simulink model "kongzhi"  (R2023a)
settings: Solver=ode23tb  StartTime=0.0  StopTime=0.5  RelTol=1e-3
libraries: spsAsynchronousMachineSIUnitsLib x1, spsDCVoltageSourceLib x1, spsGroundLib x1, spsThreePhaseVIMeasurementLib x1, spsUniversalBridgeLib x1, sps_lib x1
settings Model: Creator=ASUS  LastModifiedBy=ASUS

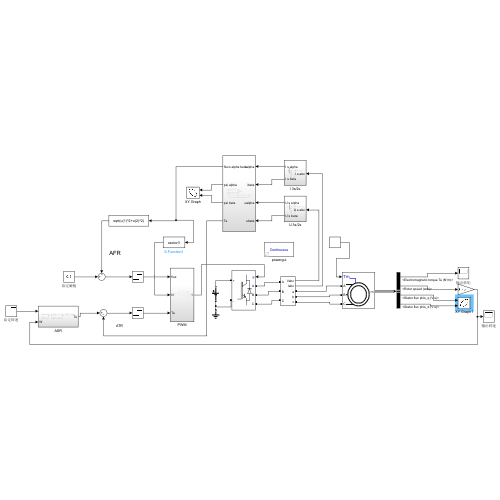
[thumbnail: Simulink's stored preview of the top-level diagram]
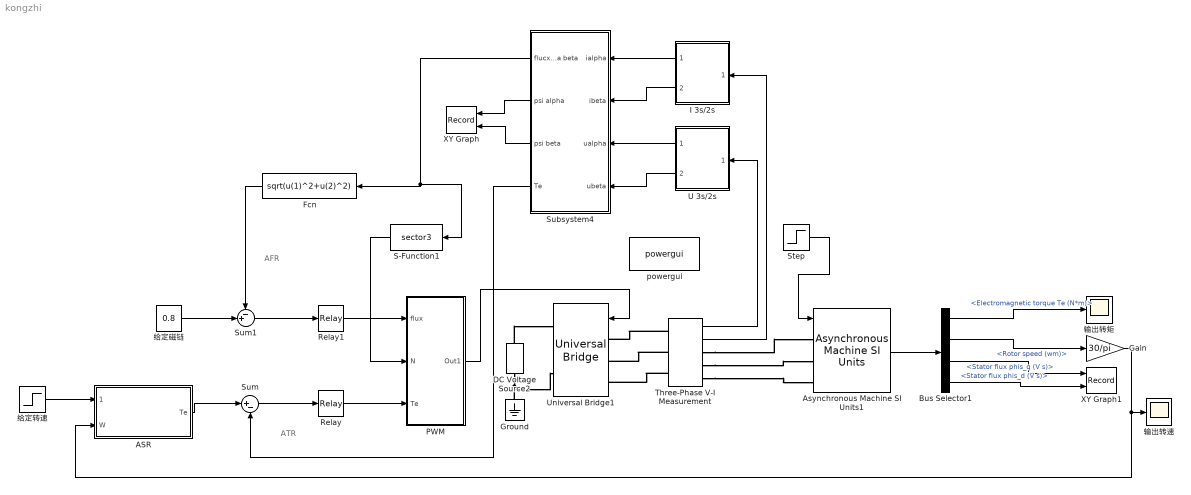
== system kongzhi ==
  note: ATR
  note: AFR
  ASR : Subsystem
  Asynchronous Machine SI Units1 : spsAsynchronousMachineSIUnitsLib/Asynchronous Machine SI Units  RotorType=Squirrel-cage  PresetModel="17:  20 HP (15KW)   400 V 50Hz 1460 RPM"  MechanicalLoad=Torque Tm  ShowDetailedParameters=on  ReferenceFrame=Stationary  Units=SI  MeasurementBus=off  NominalParameters=[1.5e+04 400 50]  VoltageRatio=1  Stator=[0.2147 0.000991]  Rotor=[0.2205 0.000991]  Cage1=[ 0.022 0.226/377]  Cage2=[ 0.022 0.226/377]  Lm=0.06419  Mechanical=[0.102 0.009541 2]  PolePairs=2  InitialConditions="[ 1,0   0,0,0   0,0,0 ]"  SimulateSaturation=off  Saturation=[9.9249,19.6672,38.0377,51.3988,69.2824,105.1337,152.5532,214.2421,303.1917;230, 322, 414, 460, 506, 552, 598, 644, 690]  LoadFlowParameters=0  TsPowergui=0  TsBlock=-1  IterativeModel=Forward Euler  IterativeDiscreteModel=Trapezoidal non iterative  Pmec=0
  Bus Selector1 : BusSelector  OutputSignals=Mechanical.Electromagnetic torque Te (N*m),Mechanical.Rotor speed (wm),Stator measurements.Stator flux phis_q (V s),Stator measurements.Stator flux phis_d (V s)
  DC Voltage Source2 : spsDCVoltageSourceLib/DC Voltage Source  Amplitude=400  Measurements=None
  Fcn : Fcn  Expr=sqrt(u(1)^2+u(2)^2)
  Gain : Gain  Gain=30/pi
  Ground : spsGroundLib/Ground  LConnTagsString=a
  I 3s/2s : Subsystem
  PWM : Subsystem
  Relay : Relay  OnSwitchValue=0.5  OffSwitchValue=-0.5
  Relay1 : Relay  OnSwitchValue=0.001  OffSwitchValue=-0.001
  S-Function1 : S-Function  FunctionName=sector3  SFunctionDeploymentMode=off  EnableBusSupport=off
  Step : Step  Time=0  Before=50  After=50  SampleTime=0
  Subsystem4 : Subsystem
  Sum : Sum  Inputs=|+-
  Sum1 : Sum  Inputs=-+|
  Three-Phase V-I Measurement : spsThreePhaseVIMeasurementLib/Three-Phase V-I Measurement  VoltageMeasurement=phase-to-ground  SetLabelV=off  LabelV=Vabc  Vpu=off  VpuLL=off  CurrentMeasurement=yes  SetLabelI=off  LabelI=Iabc  Ipu=off  Pbase=100e6  Vbase=500e3  OutputType=Complex  PhasorSimulation=off  PSBequivalent=0
  U 3s/2s : Subsystem
  Universal Bridge1 : spsUniversalBridgeLib/Universal Bridge  Arms=3  SnubberResistance=1e5  SnubberCapacitance=inf  Device=IGBT / Diodes  Ron=1e-3  Lon=0  ForwardVoltages="[  0  0  ]"  ForwardVoltage=0  GTOparameters=[ 10e-6 , 20e-6 ]  IGBTparameters=[ 1e-6 , 2e-6 ]  Measurements=None  Measurements_2=None  converterType=Rectifier
  XY Graph : Record  FileSettingsInternal="{\"entries\":[{\"content\":{\"excelSettings\":{\"content\":{},\"type\":\"Streamout.ExcelSettings\"}},\"type\":\"Streamout.FileSettingStorage\",\"uuid\":\"d99a5585-4551-4ee5-a23c-574eb21537c6\"}],\"packageUris\":[\"http://schema.mathworks.com/mf0/streamout_blocks/R2020a\"],\"version\":\"1.0\"}"  Layout=[1 1]  SignalsInternal="{\"entries\":[{\"content\":{\"signals\":[{\"content\":{\"blockPath\":[\"kongzhi/XY Graph\"],\"dimensions\":[1],\"domain\":\"kongzhi/XY Graph\",\"lineColor\":\"#a2142f\",\"plots\":[1],\"port\":1,\"sid\":[\"\"],\"signalID\":22656,\"signalName\":\"Subsystem4:2\"},\"type\":\"RecordBlkView.Signal\",\"uuid\":\"df6e7023-f9b9-436d-a626-336ee013b6ea\"},{\"content\":{\"blockPath\":[\"kongzhi/XY Graph\"],\"dimensions\":[1],\"domain\":\"kongzhi/XY Graph\",\"lineColor\":\"#139fff\",\"plots\":[1],\"port\":2,\"sid\":[\"\"],\"signalID\":22660,\"signalName\":\"Subsystem4:3\"},\"type\":\"RecordBlkView.Signal\",\"uuid\":\"d19e1cbc-f2ff-4bfc-97e4-62be1705afae\"}]},\"type\":\"RecordBlkView.InputSignals\",\"uuid\":\"3aea963f-f125-4d09-981d-9f07b36c2ba5\"}],\"packageUris\":[\"http://schema.mathworks.com/mf0/streamout_blocks/R2020a\"],\"version\":\"1.0\"}"  VisualizationBindings="{\"xyplotplugin\":{\"info\":[{\"series\":[{\"bindingParametersList\":[{\"parameter\":\"X-Axis\",\"signalID\":22656,\"signalName\":\"Subsystem4:2\"},{\"parameter\":\"Y-Axis\",\"signalID\":22660,\"signalName\":\"Subsystem4:3\"}],\"seriesID\":30182}],\"subplotID\":1}]}}"  CompatibilityTag=XY
  XY Graph1 : Record  FileSettingsInternal="{\"entries\":[{\"content\":{\"excelSettings\":{\"content\":{},\"type\":\"Streamout.ExcelSettings\"}},\"type\":\"Streamout.FileSettingStorage\",\"uuid\":\"2f48a670-b858-471d-9210-6afec38b2273\"}],\"packageUris\":[\"http://schema.mathworks.com/mf0/streamout_blocks/R2020a\"],\"version\":\"1.0\"}"  Layout=[1 1]  SignalsInternal="{\"entries\":[{\"content\":{\"signals\":[{\"content\":{\"blockPath\":[\"kongzhi/XY Graph1\"],\"dimensions\":[1],\"domain\":\"kongzhi/XY Graph1\",\"lineColor\":\"#a2142f\",\"plots\":[1],\"port\":1,\"sid\":[\"\"],\"signalID\":22664,\"signalName\":\"<Stator flux phis_q (V s)>\"},\"type\":\"RecordBlkView.Signal\",\"uuid\":\"a525e989-c708-4338-98a2-6f3b374b03e2\"},{\"content\":{\"blockPath\":[\"kongzhi/XY Graph1\"],\"dimensions\":[1],\"domain\":\"kongzhi/XY Graph1\",\"lineColor\":\"#139fff\",\"plots\":[1],\"port\":2,\"sid\":[\"\"],\"signalID\":22668,\"signalName\":\"<Stator flux phis_d (V s)>\"},\"type\":\"RecordBlkView.Signal\",\"uuid\":\"1f8a1f75-314e-4074-bfd5-83f112e8ba22\"}]},\"type\":\"RecordBlkView.InputSignals\",\"uuid\":\"839f365b-2055-442e-9575-d9756f1278d4\"}],\"packageUris\":[\"http://schema.mathworks.com/mf0/streamout_blocks/R2020a\"],\"version\":\"1.0\"}"  VisualizationBindings="{\"xyplotplugin\":{\"info\":[{\"series\":[{\"bindingParametersList\":[{\"parameter\":\"X-Axis\",\"signalID\":22664,\"signalName\":\"<Stator flux phis_q (V s)>\"},{\"parameter\":\"Y-Axis\",\"signalID\":22668,\"signalName\":\"<Stator flux phis_d (V s)>\"}],\"seriesID\":31724}],\"subplotID\":1}]}}"  CompatibilityTag=XY
  powergui : sps_lib/powergui  Priority=1  SimulationMode=Continuous  SampleTime=50e-6  frequency=60  Iterations=50  frequencyindice=50  Pbase=100e6  ErrMax=1e-4  UnitsV=kV  UnitsW=MW  buscounter=0  FunctionMessages=off  echomessages=off  EnableUseOfTLC=off  CurrentSourceSwitches=off  DisableSnubberDevices=off  DisableRonSwitches=off  DisableVfSwitches=off  DisplayEquations=off  AutomaticDiscreteSolvers=off  SolverType=Tustin/Backward Euler (TBE)  Interpol=off  ExternalGateDelay=off  methode=off  Ts=100  x0status=blocks  SPID=on  SwTol=0  HookPort=off  NonlinearTolerance=1e-4  nMaxIteration=100  ContinueOnMaxIteration=off  RestoreLinks=warning  ResistiveCurrentMeasurement=off  Frange=[0:2:500]  Ylog=off  Xlog=on  ShowGrid=off  save=off  variable=ZData  structure=0  ZoomFFT=off  StartTime=0.0  cycles=1  DisplayStyle=1  fundamental=60  FreqAxis=off  MaxFrequency=1000  frequencyindicesteady=1  RmsSteady=1  display=off
  给定磁链 : Constant  Value=0.8
  给定转速 : Step  Time=0  Before=1000  After=1000  SampleTime=0  VectorParams1D=off
  输出转矩 : Scope
  输出转速 : Scope
  wires:
  Asynchronous Machine SI Units1/1 -> Bus Selector1/1
  给定转速/1 -> ASR/1(" ")
  Bus Selector1/2 -> Gain/1  "<Rotor speed (wm)>"
  Gain/1 -> ASR/2(W), 输出转速/1
  ASR/1(Te) -> Sum/1
  Sum/1 -> Relay/1
  Sum1/1 -> Relay1/1
  Relay1/1 -> PWM/1(flux)
  Relay/1 -> PWM/3(Te)
  S-Function1/1 -> PWM/2(N)
  PWM/1(Out1) -> Universal Bridge1/1
  Three-Phase V-I Measurement/2 -> I 3s/2s/1(I s abc)
  Three-Phase V-I Measurement/1 -> U 3s/2s/1(U s abc)
  I 3s/2s/1(I s alpha) -> Subsystem4/1(ialpha)
  I 3s/2s/2(I s beta) -> Subsystem4/2(ibeta)
  U 3s/2s/1(U s alpha) -> Subsystem4/3(ualpha)
  U 3s/2s/2(U s beta) -> Subsystem4/4(ubeta)
  Subsystem4/2(psi alpha) -> XY Graph/1
  Subsystem4/3(psi beta) -> XY Graph/2
  Subsystem4/1(flucx alpha beta) -> S-Function1/1, Fcn/1
  给定磁链/1 -> Sum1/2
  Fcn/1 -> Sum1/1
  Subsystem4/4(Te) -> Sum/2
  Bus Selector1/1 -> 输出转矩/1  "<Electromagnetic torque Te (N*m)>"
  Step/1 -> Asynchronous Machine SI Units1/1
  Bus Selector1/3 -> XY Graph1/1  "<Stator flux phis_q (V s)>"
  Bus Selector1/4 -> XY Graph1/2  "<Stator flux phis_d (V s)>"
  connections:
  DC Voltage Source2/LConn1 -- Universal Bridge1/RConn2 -- Ground/LConn1
  DC Voltage Source2/RConn1 -- Universal Bridge1/RConn1
  Three-Phase V-I Measurement/LConn1 -- Universal Bridge1/LConn1
  Three-Phase V-I Measurement/LConn2 -- Universal Bridge1/LConn2
  Three-Phase V-I Measurement/LConn3 -- Universal Bridge1/LConn3
  Three-Phase V-I Measurement/RConn2 -- Asynchronous Machine SI Units1/LConn2
  Three-Phase V-I Measurement/RConn3 -- Asynchronous Machine SI Units1/LConn3
  Three-Phase V-I Measurement/RConn1 -- Asynchronous Machine SI Units1/LConn1

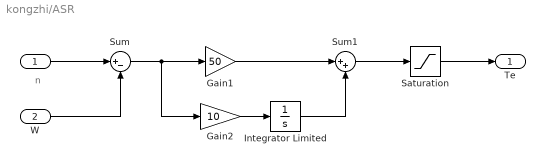
== system kongzhi/ASR ==
  note: n
  " " : Inport
  W : Inport  Port=2
  Gain1 : Gain  Gain=50
  Gain2 : Gain  Gain=10  OutMin=[-200]  OutMax=[200]
  Integrator Limited : Integrator  LimitOutput=on  UpperSaturationLimit=120  LowerSaturationLimit=-120
  Saturation : Saturate  UpperLimit=120  LowerLimit=-120
  Sum : Sum  Inputs=|+-
  Sum1 : Sum  Inputs=|++
  Te : Outport  VectorParamsAs1DForOutWhenUnconnected=off
  wires:
  Integrator Limited/1 -> Sum1/2
  " "/1 -> Sum/1
  Gain1/1 -> Sum1/1
  Sum/1 -> Gain2/1, Gain1/1
  Gain2/1 -> Integrator Limited/1
  Sum1/1 -> Saturation/1
  W/1 -> Sum/2
  Saturation/1 -> Te/1

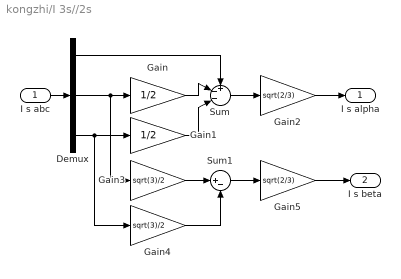
== system kongzhi/I 3s//2s ==
  I s abc : Inport
  Demux : Demux  Outputs=3
  Gain : Gain  Gain=1/2
  Gain1 : Gain  Gain=1/2
  Gain2 : Gain  Gain=sqrt(2/3)
  Gain3 : Gain  Gain=sqrt(3)/2
  Gain4 : Gain  Gain=sqrt(3)/2
  Gain5 : Gain  Gain=sqrt(2/3)
  Sum : Sum  Inputs=+--|
  Sum1 : Sum  Inputs=|+-
  I s alpha : Outport  VectorParamsAs1DForOutWhenUnconnected=off
  I s beta : Outport  Port=2  VectorParamsAs1DForOutWhenUnconnected=off
  wires:
  I s abc/1 -> Demux/1
  Demux/1 -> Sum/1
  Demux/3 -> Gain4/1, Gain1/1
  Demux/2 -> Gain3/1, Gain/1
  Sum/1 -> Gain2/1
  Gain2/1 -> I s alpha/1
  Gain3/1 -> Sum1/1
  Gain4/1 -> Sum1/2
  Sum1/1 -> Gain5/1
  Gain/1 -> Sum/2
  Gain1/1 -> Sum/3
  Gain5/1 -> I s beta/1

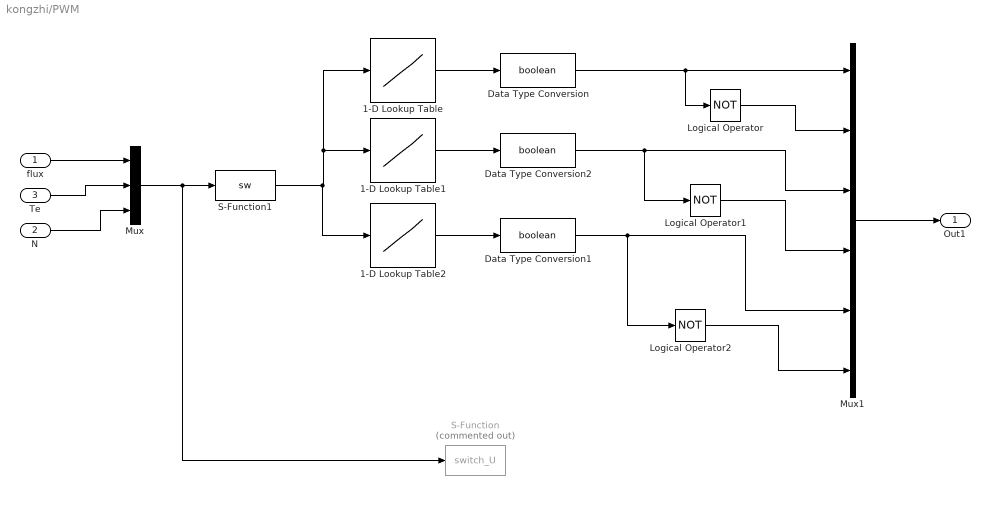
== system kongzhi/PWM ==
  flux : Inport
  N : Inport  Port=2
  Te : Inport  Port=3
  1-D Lookup Table : Lookup_n-D  NumberOfTableDimensions=1  BreakpointsForDimension1=[1 2 3 4 5 6]  Table=[1 1 1 0 0 0]  InternalRulePriority=Speed  RndMeth=Simplest
  1-D Lookup Table1 : Lookup_n-D  NumberOfTableDimensions=1  BreakpointsForDimension1=[1 2 3 4 5 6]  Table=[1 0 0 1 1 0]  InternalRulePriority=Speed  RndMeth=Simplest
  1-D Lookup Table2 : Lookup_n-D  NumberOfTableDimensions=1  BreakpointsForDimension1=[1 2 3 4 5 6]  Table=[0 1 0 1 0 1]  InternalRulePriority=Speed  RndMeth=Simplest
  Data Type Conversion : DataTypeConversion  OutDataTypeStr=boolean  SaturateOnIntegerOverflow=off  RndMeth=Floor
  Data Type Conversion1 : DataTypeConversion  OutDataTypeStr=boolean  SaturateOnIntegerOverflow=off  RndMeth=Floor
  Data Type Conversion2 : DataTypeConversion  OutDataTypeStr=boolean  SaturateOnIntegerOverflow=off  RndMeth=Floor
  Logical Operator : Logic  Operator=NOT  AllPortsSameDT=off  OutDataTypeStr=boolean
  Logical Operator1 : Logic  Operator=NOT  AllPortsSameDT=off  OutDataTypeStr=boolean
  Logical Operator2 : Logic  Operator=NOT  AllPortsSameDT=off  OutDataTypeStr=boolean
  Mux : Mux  Inputs=3
  Mux1 : Mux  Inputs=6
  S-Function : S-Function  Commented=on  FunctionName=switch_U  SFunctionDeploymentMode=off  EnableBusSupport=off
  S-Function1 : S-Function  FunctionName=sw  SFunctionDeploymentMode=off  EnableBusSupport=off
  Out1 : Outport
  wires:
  flux/1 -> Mux/1
  Te/1 -> Mux/2
  N/1 -> Mux/3
  S-Function1/1 -> 1-D Lookup Table2/1, 1-D Lookup Table1/1, 1-D Lookup Table/1
  1-D Lookup Table/1 -> Data Type Conversion/1
  1-D Lookup Table1/1 -> Data Type Conversion2/1
  1-D Lookup Table2/1 -> Data Type Conversion1/1
  Data Type Conversion/1 -> Logical Operator/1, Mux1/1
  Logical Operator/1 -> Mux1/2
  Data Type Conversion2/1 -> Logical Operator1/1, Mux1/3
  Logical Operator1/1 -> Mux1/4
  Data Type Conversion1/1 -> Logical Operator2/1, Mux1/5
  Logical Operator2/1 -> Mux1/6
  Mux/1 -> S-Function/1, S-Function1/1
  Mux1/1 -> Out1/1

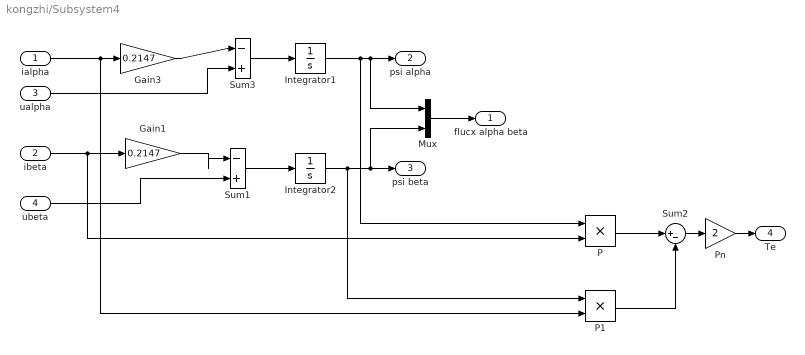
== system kongzhi/Subsystem4 ==
  ialpha : Inport
  ibeta : Inport  Port=2
  ualpha : Inport  Port=3
  ubeta : Inport  Port=4
  Gain1 : Gain  Gain=0.2147
  Gain3 : Gain  Gain=0.2147
  Integrator1 : Integrator
  Integrator2 : Integrator
  Mux : Mux  Inputs=2
  P : Product  Inputs=**
  P1 : Product  Inputs=**
  Pn : Gain  Gain=2
  Sum1 : Sum  Inputs=|-+
  Sum2 : Sum  Inputs=|+-
  Sum3 : Sum  Inputs=|-+
  flucx alpha beta : Outport
  psi alpha : Outport  Port=2
  psi beta : Outport  Port=3
  Te : Outport  Port=4  VectorParamsAs1DForOutWhenUnconnected=off
  wires:
  ialpha/1 -> P1/2, Gain3/1
  Gain3/1 -> Sum3/1
  ualpha/1 -> Sum3/2
  ubeta/1 -> Sum1/2
  ibeta/1 -> P/2, Gain1/1
  Gain1/1 -> Sum1/1
  Sum3/1 -> Integrator1/1
  Sum1/1 -> Integrator2/1
  Integrator1/1 -> P/1, Mux/1, psi alpha/1
  Mux/1 -> flucx alpha beta/1
  P/1 -> Sum2/1
  P1/1 -> Sum2/2
  Sum2/1 -> Pn/1
  Pn/1 -> Te/1
  Integrator2/1 -> P1/1, psi beta/1, Mux/2

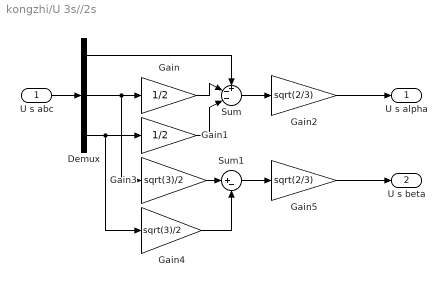
== system kongzhi/U 3s//2s ==
  U s abc : Inport
  Demux : Demux  Outputs=3
  Gain : Gain  Gain=1/2
  Gain1 : Gain  Gain=1/2
  Gain2 : Gain  Gain=sqrt(2/3)
  Gain3 : Gain  Gain=sqrt(3)/2
  Gain4 : Gain  Gain=sqrt(3)/2
  Gain5 : Gain  Gain=sqrt(2/3)
  Sum : Sum  Inputs=+--|
  Sum1 : Sum  Inputs=|+-
  U s alpha : Outport  VectorParamsAs1DForOutWhenUnconnected=off
  U s beta : Outport  Port=2  VectorParamsAs1DForOutWhenUnconnected=off
  wires:
  Demux/3 -> Gain4/1, Gain1/1
  U s abc/1 -> Demux/1
  Gain/1 -> Sum/2
  Sum1/1 -> Gain5/1
  Gain4/1 -> Sum1/2
  Gain5/1 -> U s beta/1
  Demux/2 -> Gain3/1, Gain/1
  Demux/1 -> Sum/1
  Gain2/1 -> U s alpha/1
  Gain3/1 -> Sum1/1
  Gain1/1 -> Sum/3
  Sum/1 -> Gain2/1
